simulink model "RedCrane_kinematic_model"  (R2024a)
settings: Solver=FixedStepAuto  StartTime=0.0  StopTime=8  FixedStep=Ts  MaxStep=0.005  RelTol=1e-3
values from neighbouring files (symbols this model uses):
  M = [1, 0, 0, (L5 + L4 - L1) ... (first row only)    [enviroment_setup.m]
  SList = [ws_mat ... (first row only)    [enviroment_setup.m]
  telescope0 = 4    [enviroment_setup.m]
  thetaList0 = [0, 0, 0, 0, 0]'    [enviroment_setup.m]
  Ts = 0.001    [enviroment_setup.m]
undefined symbols (not defined in the file or in its folder): p_k_angle_to_stroke, p_k_stroke_to_angle, p_m_angle_to_stroke, p_m_stroke_to_angle, X, Y, Z
libraries: sm_lib x82, nesl_utility x19, fl_lib x16
(part 1 of 3)
settings Model: Creator=sindr  LastModifiedBy=larso
settings RTWCC: GPUComputeCapability=3.5

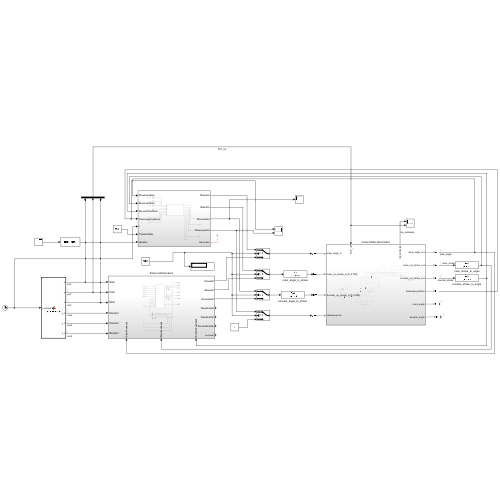
[thumbnail: Simulink's stored preview of the top-level diagram]
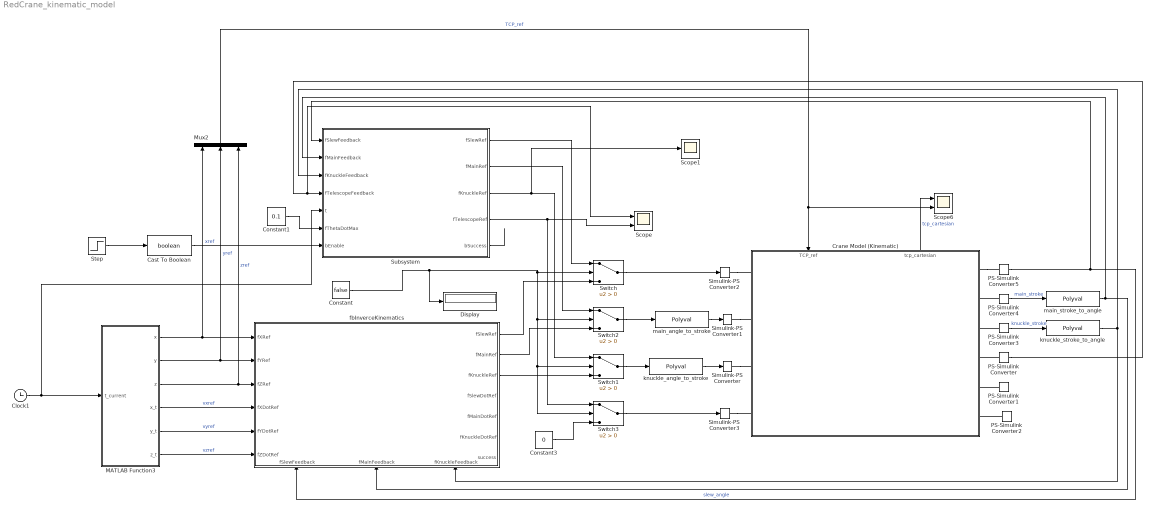
== system RedCrane_kinematic_model ==
  Cast To Boolean : DataTypeConversion  OutDataTypeStr=boolean  SaturateOnIntegerOverflow=off  RndMeth=Floor
  Clock1 : Clock
  Constant : Constant  Value=false
  Constant1 : Constant  Value=0.1
  Constant3 : Constant  Value=0
  Crane Model (Kinematic) : Subsystem
      settings: PortSchema="{\"entries\":[{\"content\":{\"sides\":[{\"content\":{\"connectorIds\":[\"LConn1\",\"LConn2\",\"LConn3\",\"LConn4\"]},\"type\":\"ConnectorPlacement.EquallySpacedRectSide\",\"uuid\":\"4a665765-5f1a-426d-91c2-f3af20fe3627\"},{\"content\":{\"connectorIds\":[\"RConn1\",\"RConn2\",\"RConn3\",\"RConn4\",\"RConn5\",\"RConn6\"],\"side\":\"RIGHT\"},\"type\":\"ConnectorPlacement.EquallySpacedRectSide\",\"uuid\":\"cf43645c-9a50-4bc9-b355-f38e72b1430d\"},{\"content\":{\"connectorIds\":[\"In1\",\"Out1\"],\"side\":\"TOP\"},\"type\":\"ConnectorPlacement.EquallySpacedRectSide\",\"uuid\":\"253dbb23-7a12-4bfe-bf07-7d8403188f09\"}]},\"type\":\"ConnectorPlacement.EquallySpacedConnector\",\"uuid\":\"5ffb1dcc-76b9-4b5c-ba8f-4653fe2f07c9\"}],\"packageUris\":[\"http://schema.mathworks.com/mf0/Connector/R2020b\"],\"version\":\"1.0\"}"
  Display : Display
  MATLAB Function3 : MATLAB Function  TreatAsAtomicUnit=on
  Mux2 : Mux  Inputs=3
  PS-Simulink Converter{,1..5} (6 alike) : nesl_utility/PS-Simulink Converter  PhysicalDomain=network_engine_domain  SubClassName=ps_output  LeftPortType=input  RightPortType=output  PseudoPeriodic=off  Frequencies=[]  VectorFormat=inherit  Unit=inherit  AffineConversion=off
  Scope : Scope  NumInputPorts=2
  Scope1 : Scope
  Scope6 : Scope  NumInputPorts=2
  Simulink-PS Converter{,1..3} (4 alike) : nesl_utility/Simulink-PS Converter  PhysicalDomain=network_engine_domain  SubClassName=ps_input  LeftPortType=input  RightPortType=output  PseudoPeriodic=off  Frequencies=[]  NoiseDistribution=none  NoiseParameters=[]  Unit=1  AffineConversion=off  FilteringAndDerivatives=filter  SimscapeFilterOrder=2  InputFilterTimeConstant=0.001  UdotUserProvided=0
  Step : Step  SampleTime=0
  Subsystem : Subsystem
  Switch{,1..3} (4 alike) : Switch  Criteria=u2 > Threshold  SaturateOnIntegerOverflow=off  InputSameDT=off
  fbInverceKinematics : Subsystem
      settings: PortSchema="{\"entries\":[{\"content\":{\"sides\":[{\"content\":{\"connectorIds\":[\"In1\",\"In2\",\"In3\",\"In4\",\"In5\",\"In6\"]},\"type\":\"ConnectorPlacement.EquallySpacedRectSide\",\"uuid\":\"b7f3f39a-cc1b-4519-b948-004466b4d293\"},{\"content\":{\"connectorIds\":[\"Out1\",\"Out2\",\"Out3\",\"Out4\",\"Out5\",\"Out6\",\"Out7\"],\"side\":\"RIGHT\"},\"type\":\"ConnectorPlacement.EquallySpacedRectSide\",\"uuid\":\"cf571c2f-2cc7-4d1d-bbc1-a75d80a0878e\"},{\"content\":{\"side\":\"TOP\"},\"type\":\"ConnectorPlacement.EquallySpacedRectSide\",\"uuid\":\"3f697bd9-7750-4474-8da5-1be48ba53c7e\"},{\"content\":{\"connectorIds\":[\"In7\",\"In8\",\"In9\"],\"side\":\"BOTTOM\"},\"type\":\"ConnectorPlacement.EquallySpacedRectSide\",\"uuid\":\"03fa0a4e-eedb-4a48-8076-446c86a2b4f7\"}]},\"type\":\"ConnectorPlacement.EquallySpacedConnector\",\"uuid\":\"6732c767-80e6-425f-b878-60bd961dd78b\"}],\"packageUris\":[\"http://schema.mathworks.com/mf0/Connector/R2020b\"],\"version\":\"1.0\"}"
  knuckle_angle_to_stroke : Polyval  Coefs=p_k_angle_to_stroke
  knuckle_stroke_to_angle : Polyval  Coefs=p_k_stroke_to_angle
  main_angle_to_stroke : Polyval  Coefs=p_m_angle_to_stroke
  main_stroke_to_angle : Polyval  Coefs=p_m_stroke_to_angle
  wires:
  Constant3/1 -> Switch3/3
  Crane Model (Kinematic)/1(tcp_cartesian) -> Scope6/1  "tcp_cartesian"
  PS-Simulink Converter4/1 -> main_stroke_to_angle/1  "main_stroke"
  PS-Simulink Converter3/1 -> knuckle_stroke_to_angle/1  "knuckle_stroke"
  main_stroke_to_angle/1 -> Subsystem/2(fMainFeedback), fbInverceKinematics/8(fMainFeedback)
  knuckle_stroke_to_angle/1 -> Subsystem/3(fKnuckleFeedback), fbInverceKinematics/9(fKnuckleFeedback)
  main_angle_to_stroke/1 -> Simulink-PS Converter1/1
  knuckle_angle_to_stroke/1 -> Simulink-PS Converter/1
  Mux2/1 -> Crane Model (Kinematic)/1(TCP_ref), Scope6/2  "TCP_ref"
  Clock1/1 -> Subsystem/5(t), MATLAB Function3/1(t_current)
  MATLAB Function3/1(x) -> Mux2/1, fbInverceKinematics/1(fXRef)  "xref"
  MATLAB Function3/2(y) -> Mux2/2, fbInverceKinematics/2(fYRef)  "yref"
  MATLAB Function3/3(z) -> Mux2/3, fbInverceKinematics/3(fZRef)  "zref"
  Switch/1 -> Simulink-PS Converter2/1
  Switch2/1 -> main_angle_to_stroke/1
  Switch1/1 -> knuckle_angle_to_stroke/1
  Switch3/1 -> Simulink-PS Converter3/1
  MATLAB Function3/4(x_t) -> fbInverceKinematics/4(fXDotRef)  "vxref"
  PS-Simulink Converter5/1 -> Subsystem/1(fSlewFeedback), fbInverceKinematics/7(fSlewFeedback)  "slew_angle"
  MATLAB Function3/5(y_t) -> fbInverceKinematics/5(fYDotRef)  "vyref"
  MATLAB Function3/6(z_t) -> fbInverceKinematics/6(fZDotRef)  "vzref"
  fbInverceKinematics/1(fSlewRef) -> Switch/3
  fbInverceKinematics/2(fMainRef) -> Switch2/3
  fbInverceKinematics/3(fKnuckleRef) -> Switch1/3
  Subsystem/5(bSuccess) -> ?
  PS-Simulink Converter/1 -> Scope/1, Subsystem/4(fTelescopeFeedback)
  Constant1/1 -> Subsystem/6(fThetaDotMax)
  Cast To Boolean/1 -> Subsystem/7(bEnable)
  Subsystem/1(fSlewRef) -> Switch/1
  Subsystem/2(fMainRef) -> Switch2/1
  Subsystem/3(fKnuckleRef) -> Scope1/1, Switch1/1
  Subsystem/4(fTelescopeRef) -> Scope/2, Switch3/1
  Step/1 -> Cast To Boolean/1
  Constant/1 -> Switch/2, Switch2/2, Switch1/2, Switch3/2, Display/1
  connections:
  Simulink-PS Converter/RConn1 -- Crane Model (Kinematic)/LConn3
  Simulink-PS Converter2/RConn1 -- Crane Model (Kinematic)/LConn1
  Simulink-PS Converter1/RConn1 -- Crane Model (Kinematic)/LConn2
  Simulink-PS Converter3/RConn1 -- Crane Model (Kinematic)/LConn4
  PS-Simulink Converter/LConn1 -- Crane Model (Kinematic)/RConn4
  PS-Simulink Converter1/LConn1 -- Crane Model (Kinematic)/RConn5
  PS-Simulink Converter2/LConn1 -- Crane Model (Kinematic)/RConn6
  PS-Simulink Converter3/LConn1 -- Crane Model (Kinematic)/RConn3
  PS-Simulink Converter4/LConn1 -- Crane Model (Kinematic)/RConn2
  Crane Model (Kinematic)/RConn1 -- PS-Simulink Converter5/LConn1
